simulink model "EV_Torque_vectoring_control"  (R2020a)
settings: Solver=VariableStepAuto  StartTime=0.0  StopTime=T  RelTol=1e-3
values from neighbouring files (symbols this model uses):
  B1 = 1.200    (= 1.2)    [TVC_Parameters.m]
  ki = 0.2    [TVC_Parameters.m]
  kp = 1    [TVC_Parameters.m]
  m = 235    [TVC_Parameters.m]
  R = 0.3    [TVC_Parameters.m]
  T = 0.5    [TVC_Parameters.m]
  Tin = 21    [TVC_Parameters.m]
  Ts = 1e-06    [TVC_Parameters.m]
undefined symbols (not defined in the file or in its folder): DiscIntNeverNeededParam
libraries: powerlib x15, simulink_extras x3, autolibshared x3, vehdynlibsteering x1, autolibshareddiff x1, autolibsharedcoupling x1
(part 2 of 2)

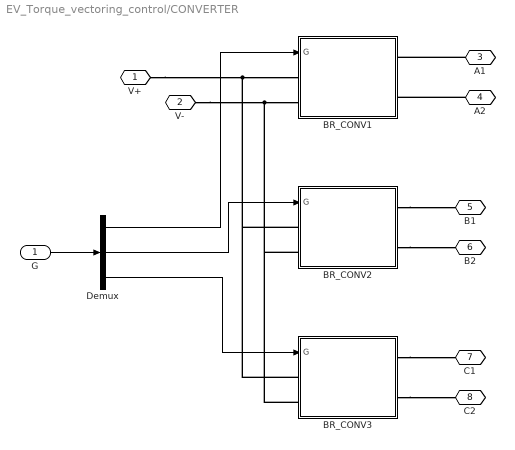
== system EV_Torque_vectoring_control/CONVERTER ==
  G : Inport
  BR_CONV1 : Subsystem
  BR_CONV2 : Subsystem
  BR_CONV3 : Subsystem
  Demux : Demux  Outputs=3
  V+ : PMIOPort  Side=Left
  V- : PMIOPort  Port=2  Side=Left
  A1 : PMIOPort  Port=3  Side=Right
  A2 : PMIOPort  Port=4  Side=Right
  B1 : PMIOPort  Port=5  Side=Right
  B2 : PMIOPort  Port=6  Side=Right
  C1 : PMIOPort  Port=7  Side=Right
  C2 : PMIOPort  Port=8  Side=Right
  wires:
  G/1 -> Demux/1
  Demux/1 -> BR_CONV1/1(G)
  Demux/2 -> BR_CONV2/1(G)
  Demux/3 -> BR_CONV3/1(G)
  connections:
  V-/RConn1 -- BR_CONV3/LConn2 -- BR_CONV2/LConn2 -- BR_CONV1/LConn2
  V+/RConn1 -- BR_CONV3/LConn1 -- BR_CONV2/LConn1 -- BR_CONV1/LConn1
  A1/RConn1 -- BR_CONV1/RConn1
  A2/RConn1 -- BR_CONV1/RConn2
  BR_CONV2/RConn1 -- B1/RConn1
  BR_CONV2/RConn2 -- B2/RConn1
  BR_CONV3/RConn1 -- C1/RConn1
  BR_CONV3/RConn2 -- C2/RConn1

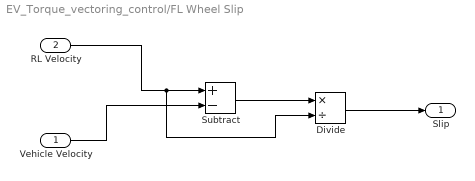
== system EV_Torque_vectoring_control/FL Wheel Slip ==
  Vehicle Velocity : Inport
  RL Velocity : Inport  Port=2
  Divide : Product  Inputs=*/
  Subtract : Sum  Inputs=+-
  "Slip " : Outport
  wires:
  Divide/1 -> "Slip "/1
  Subtract/1 -> Divide/1
  Vehicle Velocity/1 -> Subtract/2
  RL Velocity/1 -> Subtract/1, Divide/2

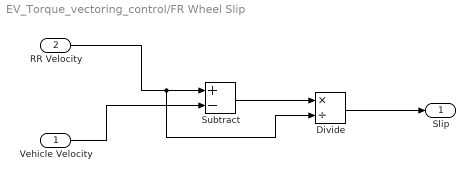
== system EV_Torque_vectoring_control/FR Wheel Slip ==
  Vehicle Velocity : Inport
  RR Velocity : Inport  Port=2
  Divide : Product  Inputs=*/
  Subtract : Sum  Inputs=+-
  Slip : Outport
  wires:
  RR Velocity/1 -> Divide/2, Subtract/1
  Vehicle Velocity/1 -> Subtract/2
  Subtract/1 -> Divide/1
  Divide/1 -> Slip/1

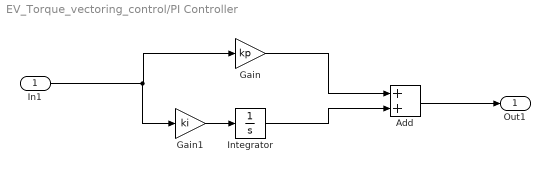
== system EV_Torque_vectoring_control/PI Controller ==
  In1 : Inport
  Add : Sum
  Gain : Gain  Gain=kp
  Gain1 : Gain  Gain=ki
  Integrator : Integrator
  Out1 : Outport
  wires:
  Gain/1 -> Add/1
  Integrator/1 -> Add/2
  In1/1 -> Gain1/1, Gain/1
  Add/1 -> Out1/1
  Gain1/1 -> Integrator/1

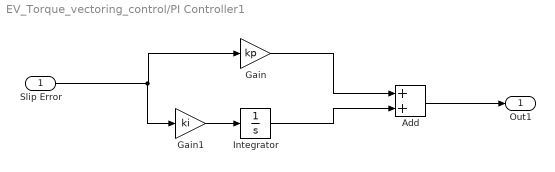
== system EV_Torque_vectoring_control/PI Controller1 ==
  Slip Error : Inport
  Add : Sum
  Gain : Gain  Gain=kp
  Gain1 : Gain  Gain=ki
  Integrator : Integrator
  Out1 : Outport
  wires:
  Add/1 -> Out1/1
  Slip Error/1 -> Gain/1, Gain1/1
  Integrator/1 -> Add/2
  Gain/1 -> Add/1
  Gain1/1 -> Integrator/1

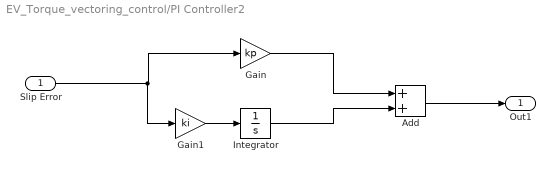
== system EV_Torque_vectoring_control/PI Controller2 ==
  Slip Error : Inport
  Add : Sum
  Gain : Gain  Gain=kp
  Gain1 : Gain  Gain=ki
  Integrator : Integrator
  Out1 : Outport
  wires:
  Gain/1 -> Add/1
  Integrator/1 -> Add/2
  Slip Error/1 -> Gain1/1, Gain/1
  Add/1 -> Out1/1
  Gain1/1 -> Integrator/1

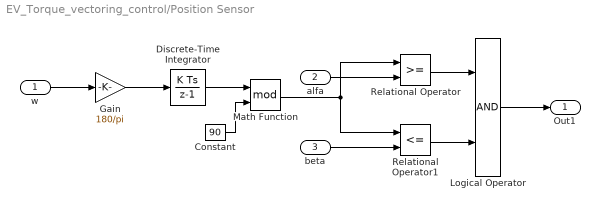
== system EV_Torque_vectoring_control/Position Sensor ==
  w : Inport
  alfa : Inport  Port=2
  beta : Inport  Port=3
  Constant : Constant  Value=90
  Discrete-Time Integrator : DiscreteIntegrator  InitialCondition=[0 -30 -60]  SampleTime=Ts  ICPrevOutput=DiscIntNeverNeededParam  ICPrevScaledInput=DiscIntNeverNeededParam
  Gain : Gain  Gain=180/pi
  Logical Operator : Logic  AllPortsSameDT=off  OutDataTypeStr=boolean
  Math Function : Math  Operator=mod  SignedPower=on  SaturateOnIntegerOverflow=on
  Relational Operator : RelationalOperator  OutDataTypeStr=boolean  RndMeth=Simplest
  Relational Operator1 : RelationalOperator  Operator=<=  OutDataTypeStr=boolean  RndMeth=Simplest
  Out1 : Outport  VectorParamsAs1DForOutWhenUnconnected=off
  wires:
  w/1 -> Gain/1
  Gain/1 -> Discrete-Time Integrator/1
  Discrete-Time Integrator/1 -> Math Function/1
  Constant/1 -> Math Function/2
  Math Function/1 -> Relational Operator/1, Relational Operator1/1
  alfa/1 -> Relational Operator/2
  beta/1 -> Relational Operator1/2
  Relational Operator/1 -> Logical Operator/1
  Relational Operator1/1 -> Logical Operator/2
  Logical Operator/1 -> Out1/1

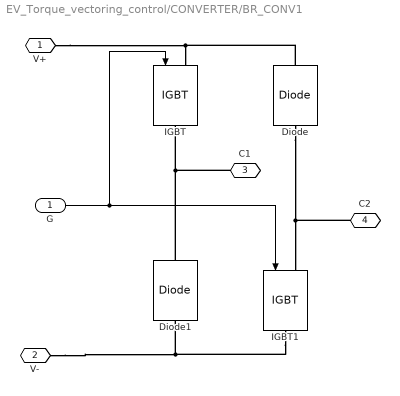
== system EV_Torque_vectoring_control/CONVERTER/BR_CONV1 ==
  G : Inport
  Diode : powerlib/Power Electronics/Diode  Ron=1E-3  Lon=0  Vf=0.8  IC=0  UseSnubber=0  Rs=1000  Cs=inf  Measurements=off
  Diode1 : powerlib/Power Electronics/Diode  Ron=1E-3  Lon=0  Vf=0.8  IC=0  UseSnubber=0  Rs=1000  Cs=inf  Measurements=off
  IGBT : powerlib/Power Electronics/IGBT  Ron=1E-3  Lon=0  Vf=1  Tf=1e-6  Tt=2e-6  IC=0  Rs=200  Cs=0.1E-06  Measurements=off
  IGBT1 : powerlib/Power Electronics/IGBT  Ron=1E-3  Lon=0  Vf=1  Tf=1e-6  Tt=2e-6  IC=0  Rs=200  Cs=0.1E-06  Measurements=off
  V+ : PMIOPort  Side=Left
  V- : PMIOPort  Port=2  Side=Left
  C1 : PMIOPort  Port=3  Side=Right
  C2 : PMIOPort  Port=4  Side=Right
  wires:
  G/1 -> IGBT1/1, IGBT/1
  connections:
  V+/RConn1 -- Diode/RConn1 -- IGBT/LConn1
  Diode/LConn1 -- C2/RConn1 -- IGBT1/LConn1
  IGBT1/RConn1 -- V-/RConn1 -- Diode1/LConn1
  Diode1/RConn1 -- C1/RConn1 -- IGBT/RConn1

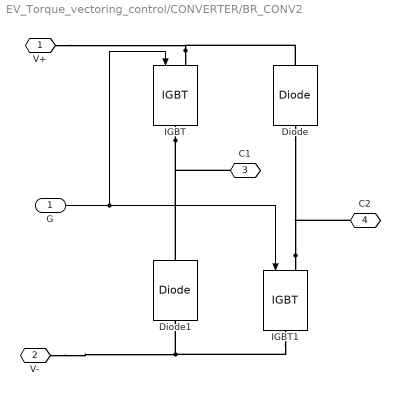
== system EV_Torque_vectoring_control/CONVERTER/BR_CONV2 ==
  G : Inport
  Diode : powerlib/Power Electronics/Diode  Ron=1E-3  Lon=0  Vf=0.8  IC=0  UseSnubber=0  Rs=1000  Cs=inf  Measurements=off
  Diode1 : powerlib/Power Electronics/Diode  Ron=1E-3  Lon=0  Vf=0.8  IC=0  UseSnubber=0  Rs=1000  Cs=inf  Measurements=off
  IGBT : powerlib/Power Electronics/IGBT  Ron=1E-3  Lon=0  Vf=1  Tf=1e-6  Tt=2e-6  IC=0  Rs=200  Cs=0.1E-06  Measurements=off
  IGBT1 : powerlib/Power Electronics/IGBT  Ron=1E-3  Lon=0  Vf=1  Tf=1e-6  Tt=2e-6  IC=0  Rs=200  Cs=0.1E-06  Measurements=off
  V+ : PMIOPort  Side=Left
  V- : PMIOPort  Port=2  Side=Left
  C1 : PMIOPort  Port=3  Side=Right
  C2 : PMIOPort  Port=4  Side=Right
  wires:
  G/1 -> IGBT1/1, IGBT/1
  connections:
  IGBT/LConn1 -- V+/RConn1 -- Diode/RConn1
  IGBT1/LConn1 -- Diode/LConn1 -- C2/RConn1
  IGBT1/RConn1 -- Diode1/LConn1 -- V-/RConn1
  IGBT/RConn1 -- Diode1/RConn1 -- C1/RConn1

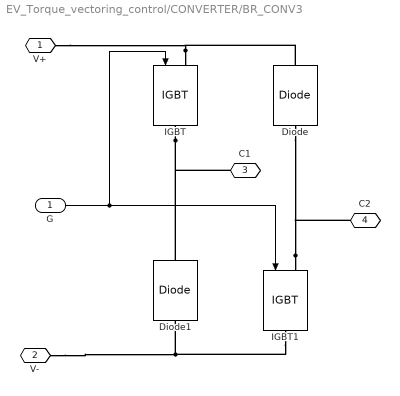
== system EV_Torque_vectoring_control/CONVERTER/BR_CONV3 ==
  G : Inport
  Diode : powerlib/Power Electronics/Diode  Ron=1E-3  Lon=0  Vf=0.8  IC=0  UseSnubber=0  Rs=1000  Cs=inf  Measurements=off
  Diode1 : powerlib/Power Electronics/Diode  Ron=1E-3  Lon=0  Vf=0.8  IC=0  UseSnubber=0  Rs=1000  Cs=inf  Measurements=off
  IGBT : powerlib/Power Electronics/IGBT  Ron=1E-3  Lon=0  Vf=1  Tf=1e-6  Tt=2e-6  IC=0  Rs=200  Cs=0.1E-06  Measurements=off
  IGBT1 : powerlib/Power Electronics/IGBT  Ron=1E-3  Lon=0  Vf=1  Tf=1e-6  Tt=2e-6  IC=0  Rs=200  Cs=0.1E-06  Measurements=off
  V+ : PMIOPort  Side=Left
  V- : PMIOPort  Port=2  Side=Left
  C1 : PMIOPort  Port=3  Side=Right
  C2 : PMIOPort  Port=4  Side=Right
  wires:
  G/1 -> IGBT1/1, IGBT/1
  connections:
  IGBT/LConn1 -- V+/RConn1 -- Diode/RConn1
  IGBT1/LConn1 -- Diode/LConn1 -- C2/RConn1
  IGBT1/RConn1 -- Diode1/LConn1 -- V-/RConn1
  IGBT/RConn1 -- Diode1/RConn1 -- C1/RConn1

== matlab function EV_Torque_vectoring_control/MATLAB Function ==
  data: u input; y output; v input; w input
function y = fcn(u,v,w)
v_r=sqrt(u^2+v^2+w^2);
y = v_r;

== matlab function EV_Torque_vectoring_control/MATLAB Function1 ==
  data: u input; y output; v input
function y = fcn(u,v)
L=4;
Rt=L*cot((u+v)/2);

y = Rt;
